simulink model "IP2"  (R2025b)
settings: Solver=VariableStepAuto  StartTime=0.0  StopTime=10  RelTol=1e-3
PostLoadFcn:
  | IP2_init
values from neighbouring files (symbols this model uses):
  A = [0, 0, 1, 0 ... (first row only)    [IP2_init.m]    (also in IP3_init.m; IP4_init.m; IP_init.m; pid_demo_init.m = [0, 0, 0)
  B = [0;0;4/ (4 * M + m); 6 / (l * (4 * M + m))]    [IP2_init.m]    (also in IP3_init.m; IP4_init.m; IP_init.m; pid_demo_init.m = [1; kd / (Tf + Ts); ki * Ts])
  C = [1, 0, 0, 0]    [IP2_init.m]    (also in IP3_init.m; IP4_init.m; IP_init.m; pid_demo_init.m = [-kd / (Tf + Ts), Tf / (Tf + Ts), 1])
  init_pos = [0, 0]    [IP2_init.m]    (also in IP3_init.m; IP4_init.m; IP_init.m; robot_velocity_input_init.m = deg2rad([0, -130, -100, -40, 90, 0]))
  K = place(A, B, p)    [IP2_init.m]    (also in IP3_init.m; IP4_init.m; IP_init.m; motor_init.m = 0.09)
  kf = -1 / (C*((A - B*K) \ B))    [IP2_init.m]    (also in IP3_init.m; IP4_init.m; IP_init.m)
  L = place(A', C', p)'    [IP2_init.m]    (also in motor_init.m = 0.0005; velocity_robot_rcm_ur5e_init.m = 0.3)
  robot = get_robot_chain(rigid_body, 'rod','base_link')    [IP2_init.m]    (also in IP3_init.m; IP4_init.m; IP_init.m; rcm_generator.m = block.DialogPrm(1).Data)
libraries: aerolibanimutils x1
settings Model: Creator=Junch  LastModifiedBy=Junch

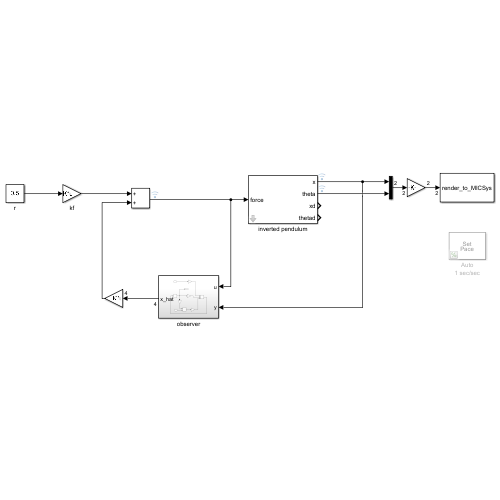
[thumbnail: Simulink's stored preview of the top-level diagram]
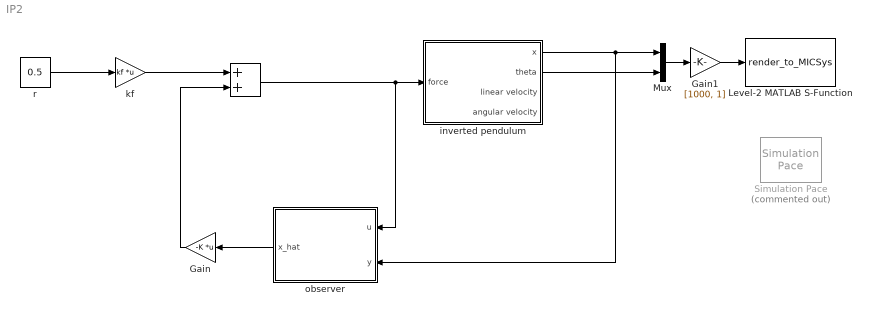
== system IP2 ==
  " " : Sum
  Gain : Gain  Gain=-K  Multiplication=Matrix(K*u)
  Gain1 : Gain  Gain=[1000, 1]
  Level-2 MATLAB S-Function : M-S-Function  FunctionName=render_to_MICSys
  Mux : Mux  Inputs=2
  Simulation Pace : aerolibanimutils/Simulation Pace  Commented=on  SimulationPace=1  SleepMode=Auto  OutputPaceError=off  SampleTime=1/30
  inverted pendulum : Subsystem  mask{robot=robot, init_pos=init_pos, Kd=[0, 0]}
      mask prompts: init_pos "intial position"; Kd "Kd (damping)"
      mask DialogControl ParameterGroupVar Prompt: 参数
      mask Display:
      | image('IP.png');
      | port_label('output', 1, 'x');
      | port_label('output', 2, 'theta');
      | port_label('output', 3, 'xd');
      | port_label('output', 4, 'thetad');
      | port_label('input', 1, 'force');
  kf : Gain  Gain=kf  Multiplication=Matrix(K*u)
  observer : Subsystem
  r : Constant  Value=0.5
  wires:
  Gain1/1 -> Level-2 MATLAB S-Function/1
  inverted pendulum/2(theta) -> Mux/2
  Mux/1 -> Gain1/1
  kf/1 -> " "/1
  r/1 -> kf/1
  " "/1 -> observer/1(u), inverted pendulum/1(force)
  inverted pendulum/1(x) -> observer/2(y), Mux/1
  observer/1(x_hat) -> Gain/1
  Gain/1 -> " "/2

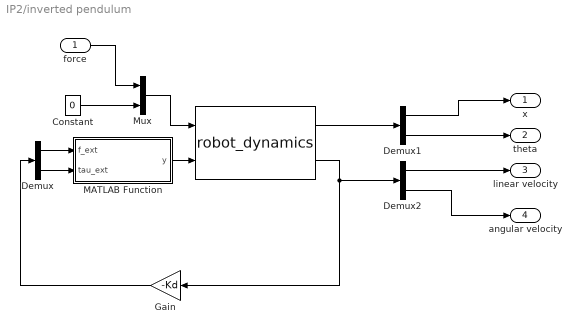
== system IP2/inverted pendulum ==
  force : Inport
  " " : M-S-Function  FunctionName=robot_dynamics  Parameters=robot, init_pos, init_vel  mask{robot=robot, init_pos=init_pos, init_vel=zeros(1,2)}
      mask prompts: robot "robot struct:"; init_pos "init pos:"; init_vel "init velocity:"
      mask DialogControl ParameterGroupVar Prompt: 参数
      mask Display:
      | port_label('input', 1, 'control torque')
      | port_label('input', 2, 'external force')
      | port_label('output', 1, 'q')
      | port_label('output', 2, 'qd')
      | disp('Robot Dynamics');
  Constant : Constant  Value=0
  Demux : Demux  Outputs=2
  Demux1 : Demux  Outputs=2
  Demux2 : Demux  Outputs=2
  Gain : Gain  Gain=-Kd
  MATLAB Function : MATLAB Function  TreatAsAtomicUnit=on
  Mux : Mux  Inputs=2
  x : Outport
  theta : Outport  Port=2
  linear velocity : Outport  Port=3
  angular velocity : Outport  Port=4
  wires:
  Demux/1 -> MATLAB Function/1(f_ext)
  Constant/1 -> Mux/2
  force/1 -> Mux/1
  Gain/1 -> Demux/1
  Mux/1 -> " "/1
  MATLAB Function/1(y) -> " "/2
  " "/2 -> Demux2/1, Gain/1
  Demux/2 -> MATLAB Function/2(tau_ext)
  " "/1 -> Demux1/1
  Demux1/1 -> x/1
  Demux1/2 -> theta/1
  Demux2/1 -> linear velocity/1
  Demux2/2 -> angular velocity/1

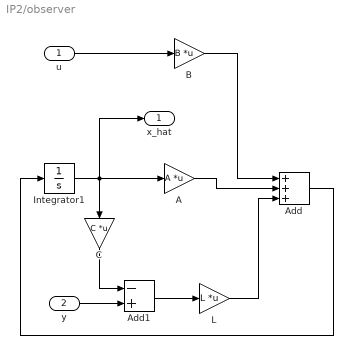
== system IP2/observer ==
  u : Inport
  y : Inport  Port=2
  A : Gain  Gain=A  Multiplication=Matrix(K*u)
  Add : Sum  Inputs=+++
  Add1 : Sum  Inputs=-+
  B : Gain  Gain=B  Multiplication=Matrix(K*u)
  C : Gain  Gain=C  Multiplication=Matrix(K*u)
  Integrator1 : Integrator
  L : Gain  Gain=L  Multiplication=Matrix(K*u)
  x_hat : Outport
  wires:
  Integrator1/1 -> x_hat/1, A/1, C/1
  u/1 -> B/1
  Add/1 -> Integrator1/1
  B/1 -> Add/1
  L/1 -> Add/3
  y/1 -> Add1/2
  Add1/1 -> L/1
  A/1 -> Add/2
  C/1 -> Add1/1

== matlab function IP2/inverted pendulum/MATLAB Function ==
  data: f_ext input; y output; tau_ext input
function y = fcn(f_ext, tau_ext)
%#codegen
y1 = [0, 0, 0, f_ext, 0, 0]';
y2 = [0, 0, tau_ext, 0, 0, 0]';
y = [y1, y2];
